simulink model "trab3_controlador"  (R2023a)
settings: Solver=VariableStepAuto  StartTime=0.0  StopTime=10.0  RelTol=1e-3
values from neighbouring files (symbols this model uses):
  A = [[-3.333 0 -1.3333];[2 -2 0];[0 4.7727 -0.04545]]    [Controlador_t3.m]    (also in lab2_controle2.m = [[0 1 0];[981.0001 0 -2.8814];[0 0 -100]]; trab3_controle2.m; trabalho1_controle2.m = [[0 1];[0 0]])
  b = [0; 0; 100]    [lab2_controle2.m]    (also in trabalho1_controle2.m = [0;-0.294])
  c = [0 0 1]    [Controlador_t3.m]    (also in lab2_controle2.m = [1 0 0]; trab3_controle2.m; trabalho1_controle2.m = [1,0])
  kii = kii*(-1)    [Controlador_t3.m]    (also in lab2_controle2.m)
  kt = place(A,b,polos_desejados)    [lab2_controle2.m]    (also in trabalho1_controle2.m)
  kt_novo_kt = vetor_k(1:3)    [Controlador_t3.m]    (also in lab2_controle2.m = kt_novo(1:3))
settings Model: Creator=wesle  LastModifiedBy=wesle

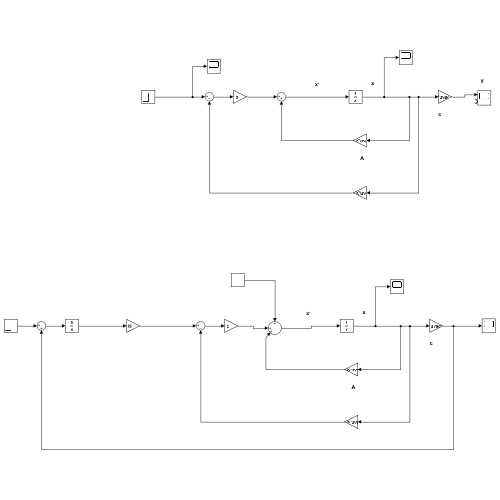
[thumbnail: Simulink's stored preview of the top-level diagram]
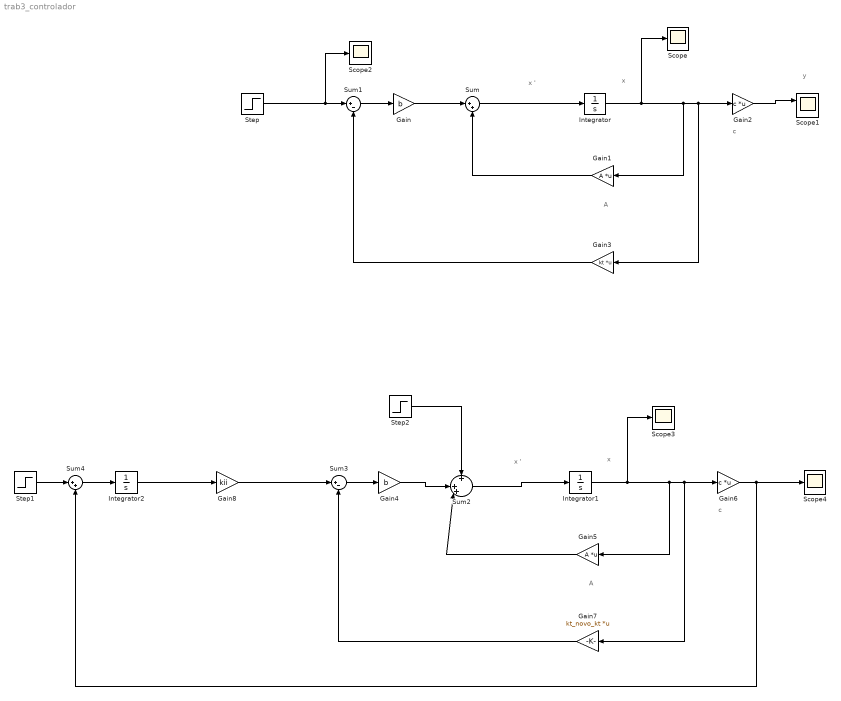
== system trab3_controlador ==
  note: c
  note: A
  note: x '
  note: x
  note: y
  note: x '
  note: A
  note: c
  note: x
  Gain : Gain  Gain=b
  Gain1 : Gain  Gain=A  Multiplication=Matrix(K*u) (u vector)
  Gain2 : Gain  Gain=c  Multiplication=Matrix(K*u) (u vector)
  Gain3 : Gain  Gain=kt  Multiplication=Matrix(K*u) (u vector)
  Gain4 : Gain  Gain=b
  Gain5 : Gain  Gain=A  Multiplication=Matrix(K*u) (u vector)
  Gain6 : Gain  Gain=c  Multiplication=Matrix(K*u) (u vector)
  Gain7 : Gain  Gain=kt_novo_kt  Multiplication=Matrix(K*u) (u vector)
  Gain8 : Gain  Gain=kii
  Integrator : Integrator
  Integrator1 : Integrator
  Integrator2 : Integrator
  Scope{,2..4} (4 alike) : Scope
  Scope1 : Scope  NumInputPorts=2
  Step : Step  After=0.0005  SampleTime=0
  Step1 : Step  After=0.0005  SampleTime=0
  Step2 : Step  Time=2.5  After=0.1  SampleTime=0
  Sum : Sum  Inputs=|++
  Sum1 : Sum  Inputs=|+-
  Sum2 : Sum  Inputs=+|++|
  Sum3 : Sum  Inputs=|+-
  Sum4 : Sum  Inputs=|++
  wires:
  Sum/1 -> Integrator/1
  Gain/1 -> Sum/1
  Gain1/1 -> Sum/2
  Step/1 -> Sum1/1, Scope2/1
  Integrator/1 -> Scope/1, Gain1/1, Gain3/1, Gain2/1
  Gain2/1 -> Scope1/1
  Gain3/1 -> Sum1/2
  Sum1/1 -> Gain/1
  Sum3/1 -> Gain4/1
  Gain7/1 -> Sum3/2
  Integrator1/1 -> Scope3/1, Gain5/1, Gain7/1, Gain6/1
  Sum2/1 -> Integrator1/1
  Gain5/1 -> Sum2/3
  Gain4/1 -> Sum2/2
  Gain6/1 -> Scope4/1, Sum4/2
  Step2/1 -> Sum2/1
  Integrator2/1 -> Gain8/1
  Step1/1 -> Sum4/1
  Sum4/1 -> Integrator2/1
  Gain8/1 -> Sum3/1
